simulink model "FLC"  (R2016b)
settings: Solver=VariableStepAuto  StartTime=0.0  StopTime=6  RelTol=1e-3
values from neighbouring files (symbols this model uses):
  A = 1.3    [PV_module_Code.m]
  Isc = 8.61    [PV_module_Code.m]
  Ki = 0.002    [PV_module_Code.m]
  Kv = -0.32    [PV_module_Code.m]
  Ns = 60    [PV_module_Code.m]
  Rp = 415    [PV_module_Code.m]
  Rs = 0.22    [PV_module_Code.m]
  Voc = 37.41    [PV_module_Code.m]
undefined symbols (not defined in the file or in its folder): sigbuilder_block
libraries: powerlib x16, powerlib_meascontrol x2, fuzblock x1
settings Model: Creator=adria  LastModifiedBy=adria

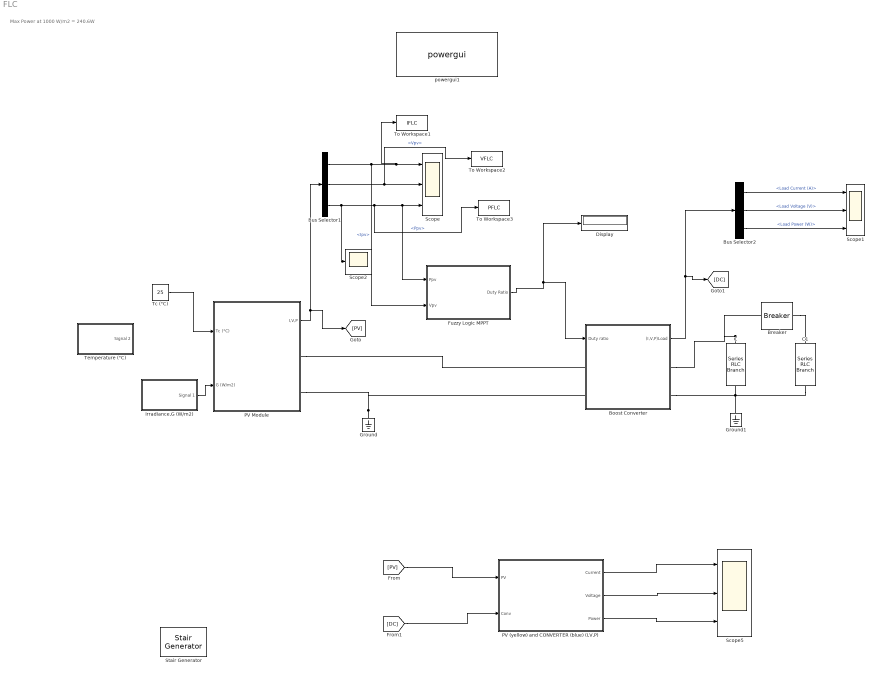
== system FLC ==
  note: Max Power at 1000 W/m2 = 240.6W
  Boost Converter : Subsystem
  Breaker : powerlib/Elements/Breaker  InitialState=0  SwitchingTimes=[5]  External=off  BreakerResistance=0.00001  SnubberResistance=1e6  SnubberCapacitance=inf  Measurements=None  MoreParameters=on  NoBreakLoop=off
  Bus Selector1 : BusSelector  OutputSignals=Ipv,Vpv,Ppv
  Bus Selector2 : BusSelector  OutputSignals=Load Current (A),Load Voltage (V),Load Power (W)
  C : powerlib/Elements/Series RLC Branch  LConnTagsString=__new0  RConnTagsString=__new0  BranchType=R  Resistance=100  Inductance=1e-3  SetiL0=off  InitialCurrent=0  Capacitance=19e-4  Setx0=off  InitialVoltage=0  Measurements=Branch voltage
  C1 : powerlib/Elements/Series RLC Branch  LConnTagsString=__new0  RConnTagsString=__new0  BranchType=R  Resistance=1000  Inductance=1e-3  SetiL0=off  InitialCurrent=0  Capacitance=19e-4  Setx0=off  InitialVoltage=0  Measurements=Branch voltage
  Display : Display
  Fuzzy Logic MPPT : Subsystem
  Ground : powerlib/Elements/Ground  LConnTagsString=a
  Ground1 : powerlib/Elements/Ground  LConnTagsString=a
  Irradiance,G (W/m2) : Subsystem  Tag=STV Subsys  LoadFcn=sigbuilder_block('load');  StartFcn=sigbuilder_block('start');  StopFcn=sigbuilder_block('stop');  ClipboardFcn=sigbuilder_block('clipboard');  mask(Sigbuilder block){tuvar=[0:10]}
      mask help: Simulink:masks:SigbuilderBlock_MD
      mask init:
      | if ~strcmp(get_param(bdroot(gcbh),'SimulationStatus'),'stopped') tuvar = sigbuilder_block('maskInit'); end
      settings: CopyFcn=sigbuilder_block('copy');  DeleteFcn=sigbuilder_block('delete');  ModelCloseFcn=sigbuilder_block('modelClose');  PreSaveFcn=sigbuilder_block('preSave');  PauseFcn=sigbuilder_block('pause');  ContinueFcn=sigbuilder_block('continue');  NameChangeFcn=sigbuilder_block('namechange');  OpenFcn=sigbuilder_block('open',[446.4 65.4 470.4 418.2 ]);  CloseFcn=sigbuilder_block('close');
      mask Display: plot(0, 0, 100, 100,[2, 2, 32, 32, 2], [68, 8, 8, 68, 68],[32, 2], [38, 38], [32, 19, 2],[53, 60, 44], [32, 17, 17, 2],[16, 16, 31, 31]);txt = getActiveGroup(gcbh);text(2, 100, txt,'verticalAlignment', 'top');
  "PV (yellow) and CONVERTER (blue) (I,V,P) " : Subsystem
  PV Module : Subsystem
  Scope : Scope  NumInputPorts=3
  Scope1 : Scope  NumInputPorts=3
  Scope2 : Scope
  Scope5 : Scope  NumInputPorts=3
  Stair Generator : powerlib_meascontrol/Pulse & Signal Generators/Stair Generator  t=[0, 0.5, 1, 1.5]  e=[700,800,900,1000]  Ts=0
  Tc (°C) : Constant  Value=25
  Temperature (°C) : Subsystem  Tag=STV Subsys  LoadFcn=sigbuilder_block('load');  StartFcn=sigbuilder_block('start');  StopFcn=sigbuilder_block('stop');  ClipboardFcn=sigbuilder_block('clipboard');  mask(Sigbuilder block){tuvar=[0:10]}
      mask help: Simulink:masks:SigbuilderBlock_MD
      mask init:
      | if ~strcmp(get_param(bdroot(gcbh),'SimulationStatus'),'stopped') tuvar = sigbuilder_block('maskInit'); end
      settings: CopyFcn=sigbuilder_block('copy');  DeleteFcn=sigbuilder_block('delete');  ModelCloseFcn=sigbuilder_block('modelClose');  PreSaveFcn=sigbuilder_block('preSave');  PauseFcn=sigbuilder_block('pause');  ContinueFcn=sigbuilder_block('continue');  NameChangeFcn=sigbuilder_block('namechange');  OpenFcn=sigbuilder_block('open',[4.8 30.6 470.4 453 ]);  CloseFcn=sigbuilder_block('close');
      mask Display: plot(0, 0, 100, 100,[2, 2, 32, 32, 2], [68, 8, 8, 68, 68],[32, 2], [38, 38], [32, 19, 2],[53, 60, 44], [32, 17, 17, 2],[16, 16, 31, 31]);txt = getActiveGroup(gcbh);text(2, 100, txt,'verticalAlignment', 'top');
  To Workspace1 : ToWorkspace  VariableName=IFLC  SampleTime=-1
  To Workspace2 : ToWorkspace  VariableName=VFLC  SampleTime=-1
  To Workspace3 : ToWorkspace  VariableName=PFLC  SampleTime=-1
  powergui1 : powerlib/powergui  Priority=1  SimulationMode=Discrete  SolverType=Tustin/Backward Euler (TBE)  SampleTime=0.000010  frequency=60  SPID=off  DisableSnubberDevices=off  DisableRonSwitches=off  DisableVfSwitches=off  SwTol=0  DisplayEquations=off  Interpol=off  ExternalGateDelay=off  methode=off  Ts=10  FunctionMessages=off  echomessages=off  HookPort=off  EnableUseOfTLC=off  x0status=blocks  frequencyindice=0  Pbase=100e6  ErrMax=1e-4  Iterations=50  UnitsV=kV  UnitsW=MW  buscounter=0  RestoreLinks=warning  ResistiveCurrentMeasurement=off  Frange=[0:2:500]  Ylog=off  Xlog=on  ShowGrid=off  save=off  variable=ZData  structure=0  ZoomFFT=off  StartTime=0.0  cycles=1  DisplayStyle=1  fundamental=60  FreqAxis=off  MaxFrequency=1000  frequencyindicesteady=1  RmsSteady=1  display=off
  wires:
  PV Module/1(I,V,P) -> [PV], Bus Selector1/1
  Bus Selector1/1 -> Fuzzy Logic MPPT/2(Vpv), To Workspace1/1, Scope/1  "<Ipv>"
  Bus Selector1/2 -> To Workspace2/1, Scope/2  "<Vpv>"
  Bus Selector1/3 -> Scope2/1, To Workspace3/1, Fuzzy Logic MPPT/1(Ppv), Scope/3  "<Ppv>"
  Bus Selector2/1 -> Scope1/1  "<Load Current (A)>"
  Bus Selector2/2 -> Scope1/2  "<Load Voltage (V)>"
  Bus Selector2/3 -> Scope1/3  "<Load Power (W)>"
  Boost Converter/1((I,V,P)Load) -> [DC], Bus Selector2/1
  [PV] -> "PV (yellow) and CONVERTER (blue) (I,V,P) "/1(PV)
  [DC] -> "PV (yellow) and CONVERTER (blue) (I,V,P) "/2(Conv)
  "PV (yellow) and CONVERTER (blue) (I,V,P) "/1(Current) -> Scope5/1
  "PV (yellow) and CONVERTER (blue) (I,V,P) "/2(Voltage) -> Scope5/2
  "PV (yellow) and CONVERTER (blue) (I,V,P) "/3(Power) -> Scope5/3
  Fuzzy Logic MPPT/1(Duty Ratio) -> Boost Converter/1("Duty ratio "), Display/1
  Tc (°C)/1 -> PV Module/1(Tc (°C))
  Irradiance,G (W/m2)/1(Signal 1) -> PV Module/2(G (W/m2))
  connections:
  Ground1/LConn1 -- Boost Converter/RConn2 -- C1/RConn1 -- C/RConn1
  Ground/LConn1 -- PV Module/RConn2 -- Boost Converter/LConn2
  C/LConn1 -- Boost Converter/RConn1 -- Breaker/LConn1
  Breaker/RConn1 -- C1/LConn1
  PV Module/RConn1 -- Boost Converter/LConn1

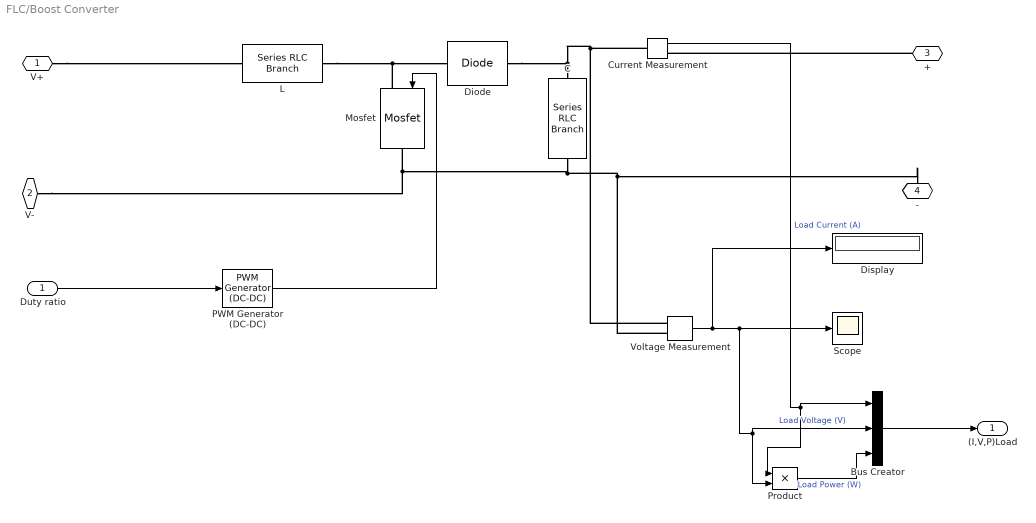
== system FLC/Boost Converter ==
  "Duty ratio " : Inport
  Bus Creator : BusCreator  Inputs='Load Current (A)','Load Voltage (V)','Load Power (W)'
  C : powerlib/Elements/Series RLC Branch  LConnTagsString=__new0  RConnTagsString=__new0  BranchType=C  Resistance=1  Inductance=1e-3  SetiL0=off  InitialCurrent=0  Capacitance=5e-5  Setx0=off  InitialVoltage=0  Measurements=None
  Current Measurement : powerlib/Measurements/Current Measurement  PhasorSimulation=off  OutputType=Complex  PSBequivalent=0
  Diode : powerlib/Power Electronics/Diode  Ron=0.0001  Lon=0  Vf=0.8  IC=0  UseSnubber=off  Rs=500  Cs=250e-9  Measurements=off
  Display : Display
  L : powerlib/Elements/Series RLC Branch  LConnTagsString=__new0  RConnTagsString=__new0  BranchType=L  Resistance=1  Inductance=1e-3  SetiL0=off  InitialCurrent=0  Capacitance=1e-6  Setx0=off  InitialVoltage=0  Measurements=None
  Mosfet : powerlib/Power Electronics/Mosfet  Ron=0.0001  Lon=0  Rd=0.0001  Vfd=0  IC=0  Rs=1e5  Cs=inf  Measurements=off
  PWM Generator (DC-DC) : powerlib_meascontrol/Pulse & Signal Generators/PWM Generator (DC-DC)  Fsw=20000  Ts=0
  Product : Product
  Scope : Scope
  Voltage Measurement : powerlib/Measurements/Voltage Measurement  PhasorSimulation=off  OutputType=Complex  PSBequivalent=0
  V+ : PMIOPort  Port=1  Side=Left
  V- : PMIOPort  Port=2  Side=Left
  + : PMIOPort  Port=3  Side=Right
  - : PMIOPort  Port=4  Side=Right
  (I,V,P)Load : Outport
  wires:
  PWM Generator (DC-DC)/1 -> Mosfet/1
  Voltage Measurement/1 -> Display/1, Product/2, Bus Creator/2, Scope/1  "Load Voltage (V)"
  "Duty ratio "/1 -> PWM Generator (DC-DC)/1
  Current Measurement/1 -> Product/1, Bus Creator/1  "Load Current (A)"
  Product/1 -> Bus Creator/3  "Load Power (W)"
  Bus Creator/1 -> (I,V,P)Load/1
  connections:
  V+/RConn1 -- L/LConn1
  L/RConn1 -- Mosfet/LConn1 -- Diode/LConn1
  +/RConn1 -- Current Measurement/RConn1
  -/RConn1 -- Voltage Measurement/LConn2 -- V-/RConn1 -- Mosfet/RConn1 -- C/RConn1
  Diode/RConn1 -- Current Measurement/LConn1 -- Voltage Measurement/LConn1 -- C/LConn1

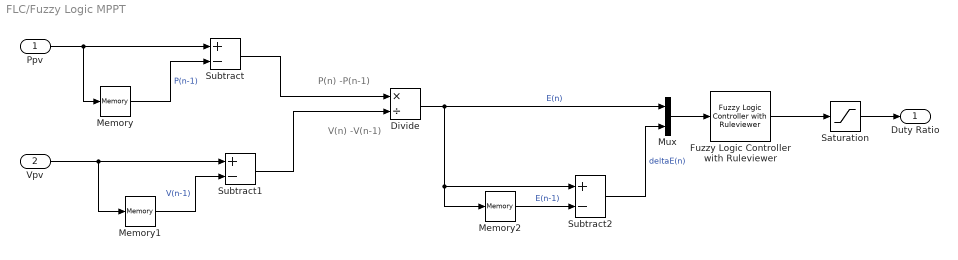
== system FLC/Fuzzy Logic MPPT ==
  note: P(n) -P(n-1)
  note: V(n) -V(n-1)
  Ppv : Inport
  Vpv : Inport  Port=2
  Divide : Product  Inputs=*/
  Fuzzy Logic Controller with Ruleviewer : fuzblock/Fuzzy Logic  Controller  with Ruleviewer  fismatrix=MPPT9  Ts=1
  Memory : Memory  InheritSampleTime=on  LinearizeMemory=on  LinearizeAsDelay=on
  Memory1 : Memory  InheritSampleTime=on  LinearizeMemory=on  LinearizeAsDelay=on
  Memory2 : Memory
  Mux : Mux  Inputs=2
  Saturation : Saturate  UpperLimit=1  LowerLimit=0.0001  LinearizeAsGain=off
  Subtract : Sum  Inputs=+-
  Subtract1 : Sum  Inputs=+-
  Subtract2 : Sum  Inputs=+-
  Duty Ratio : Outport
  wires:
  Ppv/1 -> Subtract/1, Memory/1
  Mux/1 -> Fuzzy Logic Controller with Ruleviewer/1
  Divide/1 -> Subtract2/1, Memory2/1, Mux/1  "E(n)"
  Memory2/1 -> Subtract2/2  "E(n-1)"
  Subtract2/1 -> Mux/2  "deltaE(n)"
  Memory/1 -> Subtract/2  "P(n-1)"
  Vpv/1 -> Memory1/1, Subtract1/1
  Memory1/1 -> Subtract1/2  "V(n-1)"
  Saturation/1 -> Duty Ratio/1
  Subtract1/1 -> Divide/2
  Subtract/1 -> Divide/1
  Fuzzy Logic Controller with Ruleviewer/1 -> Saturation/1

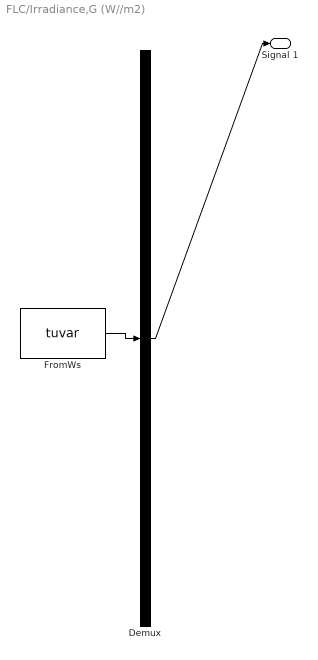
== system FLC/Irradiance,G (W//m2) ==
  Demux : Demux  Tag=STV Demux  Outputs=1
  FromWs : FromWorkspace  Tag=STV FromWs  VariableName=tuvar  SampleTime=0
      SigBuilderData=|
      | common.afterFinalStr = 'Extrapolate'
      | common.sampleTime = 0
      | dataSet.timeRange = [0 10]
      | dataSet.name = 'Irradiance Variation Pattern'
      | sbobj.Groups.Name = 'Irradiance Variation Pattern'
      | sbobj.Groups.Signals.Name = 'Signal 1'
      | sbobj.Groups.Signals.XData = [0 0.5 0.5 1 1 1.5 1.98 2.5 3 3.5 4 4.5 4.5 5 5.05 6 10]
      | sbobj.Groups.Signals.YData = [1000 1000 800 800 500 500 300 100 100 300 500 500 1000 1000 1000 1000 1000]
  Signal 1 : Outport  Tag=STV Outport
  wires:
  FromWs/1 -> Demux/1
  Demux/1 -> Signal 1/1

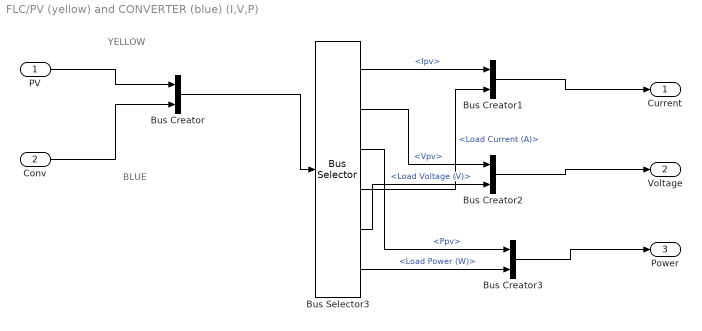
== system FLC/PV (yellow) and CONVERTER (blue) (I,V,P)  ==
  note: YELLOW
  note: BLUE
  PV : Inport
  Conv : Inport  Port=2
  Bus Creator : BusCreator  Inputs=2
  Bus Creator1 : BusCreator  Inputs='Ipv','Load Current (A)'
  Bus Creator2 : BusCreator  Inputs=2
  Bus Creator3 : BusCreator  Inputs=2
  Bus Selector3 : BusSelector  OutputSignals=signal1.Ipv,signal1.Vpv,signal1.Ppv,signal2.Load Current (A),signal2.Load Voltage (V),signal2.Load Power (W)
  Current : Outport
  Voltage : Outport  Port=2
  Power : Outport  Port=3
  wires:
  Bus Creator/1 -> Bus Selector3/1
  Bus Selector3/1 -> Bus Creator1/1  "<Ipv>"
  Bus Creator1/1 -> Current/1
  PV/1 -> Bus Creator/1
  Bus Creator2/1 -> Voltage/1
  Bus Creator3/1 -> Power/1
  Bus Selector3/4 -> Bus Creator1/2  "<Load Current (A)>"
  Bus Selector3/2 -> Bus Creator2/1  "<Vpv>"
  Conv/1 -> Bus Creator/2
  Bus Selector3/3 -> Bus Creator3/1  "<Ppv>"
  Bus Selector3/5 -> Bus Creator2/2  "<Load Voltage (V)>"
  Bus Selector3/6 -> Bus Creator3/2  "<Load Power (W)>"

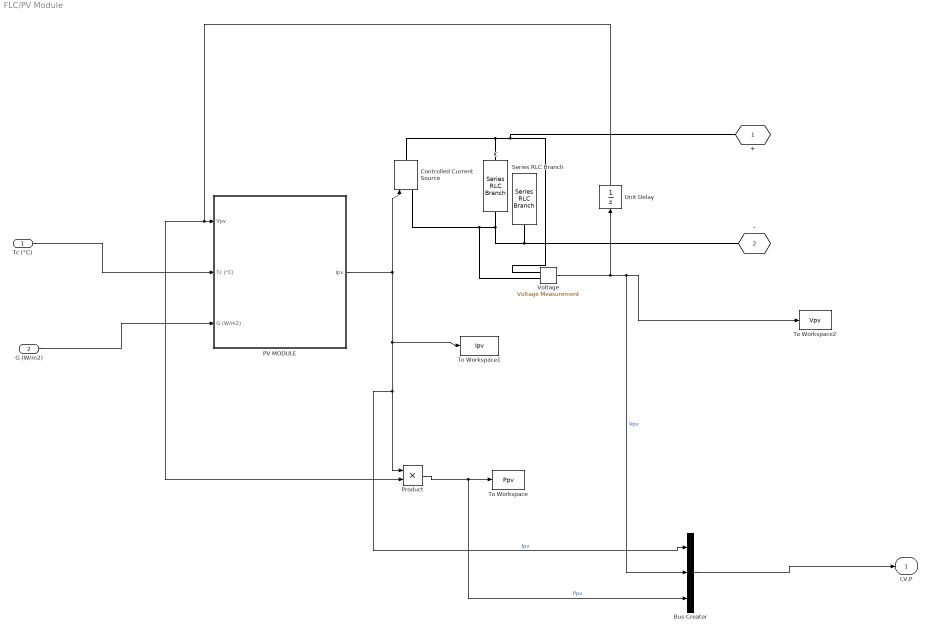
== system FLC/PV Module ==
  Tc (°C) : Inport
  G (W/m2) : Inport  Port=2
  Bus Creator : BusCreator  Inputs='Ipv','Vpv','Ppv'
  C : powerlib/Elements/Series RLC Branch  LConnTagsString=__new0  RConnTagsString=__new0  BranchType=C  Resistance=10  Inductance=1e-3  SetiL0=off  InitialCurrent=0  Capacitance=30e-4  Setx0=off  InitialVoltage=0  Measurements=Branch voltage
  Controlled Current Source : powerlib/Electrical Sources/Controlled Current Source  Initialize=on  Source_Type=DC  Amplitude=0  Phase=0  Frequency=0  Measurements=None
  PV MODULE : Subsystem
  Product : Product
  Series RLC Branch : powerlib/Elements/Series RLC Branch  LConnTagsString=__new0  RConnTagsString=__new0  BranchType=R  Resistance=1000  Inductance=1e-3  SetiL0=off  InitialCurrent=0  Capacitance=1e-6  Setx0=off  InitialVoltage=0  Measurements=None
  To Workspace : ToWorkspace  VariableName=Ppv  SampleTime=-1
  To Workspace1 : ToWorkspace  VariableName=Ipv  SampleTime=-1
  To Workspace2 : ToWorkspace  VariableName=Vpv  SampleTime=-1
  Unit Delay : UnitDelay  SampleTime=-1
  "Voltage " : powerlib/Measurements/Voltage Measurement  PhasorSimulation=off  OutputType=Complex  PSBequivalent=0
  + : PMIOPort  Port=1  Side=Right
  - : PMIOPort  Port=2  Side=Right
  I,V,P : Outport
  wires:
  Product/1 -> Bus Creator/3, To Workspace/1  "Ppv"
  Tc (°C)/1 -> PV MODULE/2("Tc (°C) ")
  G (W/m2)/1 -> PV MODULE/3(G (W/m2))
  "Voltage "/1 -> Unit Delay/1, Bus Creator/2, To Workspace2/1  "Vpv"
  PV MODULE/1(Ipv) -> Controlled Current Source/1, To Workspace1/1, Bus Creator/1, Product/1  "Ipv"
  Bus Creator/1 -> I,V,P/1
  Unit Delay/1 -> Product/2, PV MODULE/1(Vpv)
  connections:
  Controlled Current Source/LConn1 -- Series RLC Branch/RConn1 -- -/RConn1 -- C/RConn1 -- "Voltage "/LConn2
  Controlled Current Source/RConn1 -- C/LConn1 -- "Voltage "/LConn1 -- +/RConn1

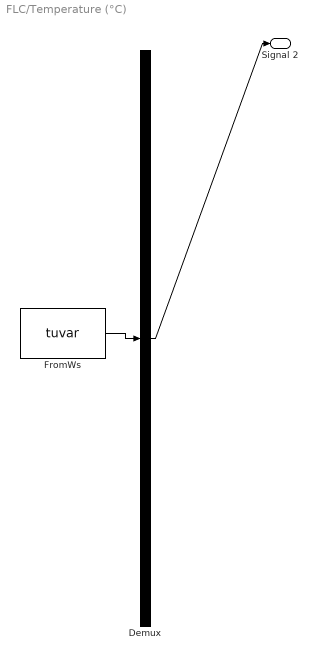
== system FLC/Temperature (°C) ==
  Demux : Demux  Tag=STV Demux  Outputs=1
  FromWs : FromWorkspace  Tag=STV FromWs  VariableName=tuvar  SampleTime=0
      SigBuilderData=|
      | common.afterFinalStr = 'Extrapolate'
      | common.sampleTime = 0
      | dataSet.timeRange = [0 10]
      | dataSet.name = 'Temperature (°C'
      | sbobj.Groups.Name = 'Temperature (°C'
      | sbobj.Groups.Signals.Name = 'Signal 2'
      | sbobj.Groups.Signals.XData = [0 0.5 0.5 1 2 2.5 3 4 4 5 9.08 9.08 10]
      | sbobj.Groups.Signals.YData = [25 25 10 10 0 0 15 45 45.2 45 45 19 19]
  Signal 2 : Outport  Tag=STV Outport
  wires:
  FromWs/1 -> Demux/1
  Demux/1 -> Signal 2/1

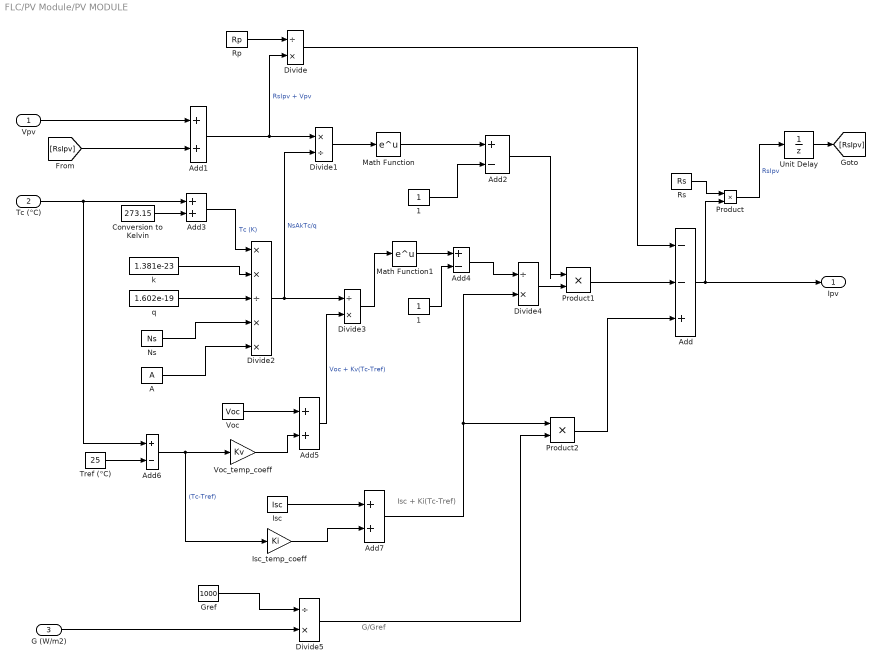
== system FLC/PV Module/PV MODULE ==
  note: G/Gref
  note: Isc + Ki(Tc-Tref)
  Vpv : Inport
  "Tc (°C) " : Inport  Port=2
  G (W/m2) : Inport  Port=3
  " 1" : Constant
  " Gref " : Constant  Value=1000
  " Tref (°C)" : Constant  Value=25
  " Voc" : Constant  Value=Voc
  1 : Constant
  A : Constant  Value=A
  Add : Sum  Inputs=--+
  Add{1,3,5,7} (4 alike) : Sum
  Add2 : Sum  Inputs=+-
  Add4 : Sum  Inputs=+-
  Add6 : Sum  Inputs=+-
  Conversion to Kelvin : Constant  Value=273.15
  Divide{,3..5} (4 alike) : Product  Inputs=/*
  Divide1 : Product  Inputs=*/
  Divide2 : Product  Inputs=**/**
  Isc : Constant  Value=Isc
  "Isc_temp_coeff " : Gain  Gain=Ki
  Math Function : Math  SaturateOnIntegerOverflow=on
  Math Function1 : Math  SaturateOnIntegerOverflow=on
  Ns : Constant  Value=Ns
  Product : Product
  Product1 : Product
  Product2 : Product
  Rp : Constant  Value=Rp
  Rs : Constant  Value=Rs
  Unit Delay : UnitDelay  SampleTime=-1
  Voc_temp_coeff : Gain  Gain=Kv
  k : Constant  Value=1.381e-23
  "q " : Constant  Value=1.602e-19
  Ipv : Outport
  wires:
  A/1 -> Divide2/5
  Vpv/1 -> Add1/1
  Rp/1 -> Divide/1
  Add/1 -> Ipv/1, Product/2
  Product/1 -> Unit Delay/1  "RsIpv"
  Divide/1 -> Add/1
  Add1/1 -> Divide1/1, Divide/2  "RsIpv + Vpv"
  Rs/1 -> Product/1
  Product2/1 -> Add/3
  Divide2/1 -> Divide3/1, Divide1/2  "NsAkTc/q"
  k/1 -> Divide2/2
  Math Function1/1 -> Add4/1
  " Voc"/1 -> Add5/1
  Divide4/1 -> Product1/2
  Add2/1 -> Product1/1
  Math Function/1 -> Add2/1
  Divide3/1 -> Math Function1/1
  "q "/1 -> Divide2/3
  Add6/1 -> "Isc_temp_coeff "/1, Voc_temp_coeff/1  "(Tc-Tref)"
  " 1"/1 -> Add4/2
  Isc/1 -> Add7/1
  Add7/1 -> Product2/1, Divide4/2
  "Tc (°C) "/1 -> Add6/1, Add3/1
  Add4/1 -> Divide4/1
  Product1/1 -> Add/2
  Divide5/1 -> Product2/2
  Conversion to Kelvin/1 -> Add3/2
  Add5/1 -> Divide3/2  "Voc + Kv(Tc-Tref)"
  "Isc_temp_coeff "/1 -> Add7/2
  Divide1/1 -> Math Function/1
  " Gref "/1 -> Divide5/1
  " Tref (°C)"/1 -> Add6/2
  G (W/m2)/1 -> Divide5/2
  Voc_temp_coeff/1 -> Add5/2
  Add3/1 -> Divide2/1  "Tc (K)"
  Ns/1 -> Divide2/4
  1/1 -> Add2/2
  [RsIpv] -> Add1/2
  Unit Delay/1 -> [RsIpv]
